simulink model "SF104A_MotCurrRegCfg"  (R2013b)
settings: Solver=FixedStepDiscrete  SolverMode=SingleTasking  StartTime=0.0  StopTime=1  FixedStep=0.002  RelTol=1e-3
values from neighbouring files (symbols this model uses):
  ARCHGLBPRM_2MILLISEC_SEC_F32 = DataDict.Constant    [SF104A_MotCurrRegCfg_DataDict.m]
  ARCHGLBPRM_2PI_ULS_F32 = DataDict.Constant    [SF104A_MotCurrRegCfg_DataDict.m]
  ARCHGLBPRM_HALFSQRT3_ULS_F32 = DataDict.Constant    [SF104A_MotCurrRegCfg_DataDict.m]
  MotCurrRegCfgCtrlrDynGainVehSpdCutOff = DataDict.Calibration    [SF104A_MotCurrRegCfg_DataDict.m]
  MotCurrRegCfgCurrLoopSecOrderTrfFctEna = DataDict.Calibration    [SF104A_MotCurrRegCfg_DataDict.m]
  MotCurrRegCfgIntglGainSampleTi = DataDict.Calibration    [SF104A_MotCurrRegCfg_DataDict.m]
  MotCurrRegCfgMotAgCompuDly = DataDict.Calibration    [SF104A_MotCurrRegCfg_DataDict.m]
  MotCurrRegCfgMotClsdLoopBwDaxY = DataDict.Calibration    [SF104A_MotCurrRegCfg_DataDict.m]
  MotCurrRegCfgMotClsdLoopBwQaxY = DataDict.Calibration    [SF104A_MotCurrRegCfg_DataDict.m]
  MotCurrRegCfgMotDampgRatDax = DataDict.Calibration    [SF104A_MotCurrRegCfg_DataDict.m]
  MotCurrRegCfgMotDampgRatQax = DataDict.Calibration    [SF104A_MotCurrRegCfg_DataDict.m]
  MotCurrRegCfgMotNatFrqDaxY = DataDict.Calibration    [SF104A_MotCurrRegCfg_DataDict.m]
  MotCurrRegCfgMotNatFrqQaxY = DataDict.Calibration    [SF104A_MotCurrRegCfg_DataDict.m]
  MotCurrRegCfgMotRVirtDax = DataDict.Calibration    [SF104A_MotCurrRegCfg_DataDict.m]
  MotCurrRegCfgMotRVirtQax = DataDict.Calibration    [SF104A_MotCurrRegCfg_DataDict.m]
  MOTDAMPGRATCON_ULS_F32 = DataDict.Constant    [SF104A_MotCurrRegCfg_DataDict.m]
  MotRefMdlFbCtrlDi = DataDict.ImprtdCal    [SF104A_MotCurrRegCfg_DataDict.m]
  POLETOPHA_ULS_F32 = DataDict.Constant    [SF104A_MotCurrRegCfg_DataDict.m]
  SysGlbPrmMotPoleCnt = DataDict.ImprtdCal    [SF104A_MotCurrRegCfg_DataDict.m]
  ZEROMOTCTRLGAIN_OHM_F32 = DataDict.Constant    [SF104A_MotCurrRegCfg_DataDict.m]
undefined symbols (not defined in the file or in its folder): MotCurrEolCalSt2
libraries: NxtrLim x11, FixdToFloat x4, LnrIntrpn x4, simulink x3, Fil x2, FloatToFixd x1
(part 1 of 3)
settings Model: Creator=qzwc4r  LastModifiedBy=RZ2YLP
settings SolverCC: AutoInsertRateTranBlk=on  InsertRTBMode=Always
settings DataIOCC: LimitDataPoints=off  SaveFormat=Structure  ReturnWorkspaceOutputs=on
settings OptimizationCC: BlockReduction=off  InlineParams=on  ZeroExternalMemoryAtStartup=off  ZeroInternalMemoryAtStartup=off  OptimizeModelRefInitCode=on  LifeSpan=1
settings DebuggingCC: SignalInfNanChecking=error  SignalRangeChecking=warning  UnderspecifiedInitializationDetection=Simplified  SolverPrmCheckMsg=error  InheritedTsInSrcMsg=error  DiscreteInheritContinuousMsg=error  SingleTaskRateTransMsg=error  TasksWithSamePriorityMsg=error  SigSpecEnsureSampleTimeMsg=error  CheckMatrixSingularityMsg=error  ParameterUnderflowMsg=error  ParameterPrecisionLossMsg=error  ParameterTunabilityLossMsg=error  FixptConstUnderflowMsg=warning  FixptConstOverflowMsg=warning  VectorMatrixConversionMsg=error  SignalLabelMismatchMsg=error  UnconnectedInputMsg=error  UnconnectedOutputMsg=error  UnconnectedLineMsg=error  SFcnCompatibilityMsg=error  UniqueDataStoreMsg=warning  BusObjectLabelMismatch=error  RootOutportRequireBusObject=error  AssertControl=DisableAll  ModelReferenceIOMsg=error  ModelReferenceVersionMismatchMessage=warning  ModelReferenceIOMismatchMessage=error  ModelReferenceCSMismatchMessage=warning  ModelReferenceDataLoggingMessage=error  StateNameClashWarn=warning  StrictBusMsg=ErrorOnBusTreatedAsVector  NonBusSignalsTreatedAsBus=error  SFUnexpectedBacktrackingDiag=error  SFInvalidInputDataAccessInChartInitDiag=error  SFNoUnconditionalDefaultTransitionDiag=error  SFTransitionOutsideNaturalParentDiag=error  SFUnconditionalTransitionShadowingDiag=error  SFUndirectedBroadcastEventsDiag=error
settings ModelReferenceCC: ModelReferenceNumInstancesAllowed=Single
settings RTWCC: SystemTargetFile=autosar.tlc  GenCodeOnly=on  TemplateMakefile=ert_default_tmf  Description=AUTOSAR  GenerateReport=on  ProcessScript=autosar_make_rtw_hook  LaunchReport=on
settings CodeAppCC: GenerateComments=off  IgnoreCustomStorageClasses=off  CustomSymbolStrType=$N$R$M  CustomSymbolStrBlkIO=$N$M  SimulinkBlockComments=off
settings STFCustomTargetCC: ParMdlRefBuildCompliant=on  CompOptLevelCompliant=on  IncludeMdlTerminateFcn=off  CombineOutputUpdateFcns=on  SuppressErrorStatus=on  ERTFirstTimeCompliant=on  ERTCustomFileBanners=on  SupportNonFinite=off  SupportComplex=off  SupportContinuousTime=off  SupportNonInlinedSFcns=off  MATLABClassNameForMDSCustomization=Simulink.SoftwareTarget.ERTCustomization  AutosarCompliant=on  GRTInterface=off  SystemTargetFile=autosar.tlc
settings ERTTargetCC: CodeReplacementLibrary=ANSI_C  ConcurrentExecutionCompliant=off  IncludeMdlTerminateFcn=off  SuppressErrorStatus=on  SupportNonFinite=off  SupportComplex=off  ModelStepFunctionPrototypeControlCompliant=off  CPPClassGenCompliant=off  AutosarCompliant=on  InlinedParameterPlacement=NonHierarchical  ERTCustomFileTemplate=example_file_process.tlc  EnableUserReplacementTypes=on

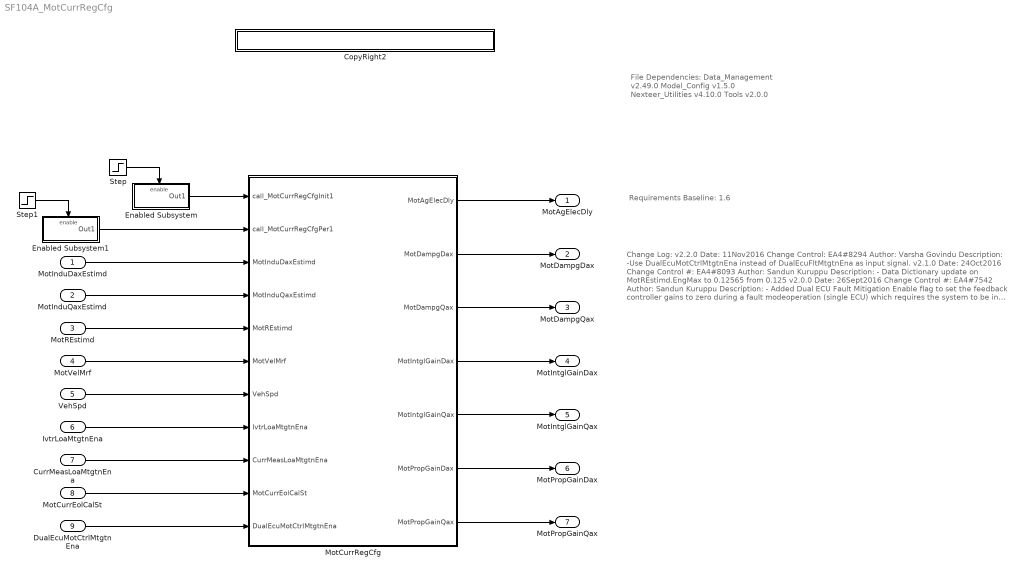
== system SF104A_MotCurrRegCfg ==
  note: File Dependencies:
      |
      | Data_Management v2.49.0
      | Model_Config v1.5.0
      | Nexteer_Utilities v4.10.0
      | Tools v2.0.0
  note: Requirements Baseline: 1.6
  note: Change Log:
      | v2.2.0
      | Date: 11Nov2016
      | Change Control: EA4#8294
      | Author: Varsha Govindu
      | Description:
      | -Use DualEcuMotCtrlMtgtnEna instead of DualEcuFltMtgtnEna as input signal.
      |
      | v2.1.0
      | Date: 24Oct2016
      | Change Control #: EA4#8093
      | Author: Sandun Kuruppu
      | Description:
      |  - Data Dictionary update on MotREstimd.EngMax to 0.12565 from 0.125
      |
      | v2.0.0
      | Date: 26Sept2016
      | Change Control #: EA4#7542
      | Author: Sandun Kuruppu
      | Description:
      | - Added Dual ECU Fault Mitigation Enable flag to set the feedback controller gains to
      | zero during a fault modeoperation (single ECU) which requires the system to be in feedforward
      | control mode
      |
      | v1.5.0
      | Date: 06Jun2016
      | Change Control #: EA4#6007
      | Author: Siva
      | Description:
      | - Updated the test tolerance value of 'MotIntglGainQax' and
      |    'MotIntglGainDax' from '1.49e-8' to '1.49e-7'.
      |
      |
      | v1.4.1
      | Date: 29April2016
      | Change Control #: EA4#5365
      | Author:  Siva
      | Description:
      | - HIghlighted only those blocks related to v1.4.0
      |
      |
      | v1.4.0
      | Date: 29April2016
      | Change Control #: EA4#5365
      | Author:  Siva
      | Description:
      | - Input signal name changed from 'MotCurrLoaMtgtnEna' to 'CurrMeasLoaMtgtnEna'.
      |
      |
      | v1.3.0
      | Date: 16November2015
      | Change Control #: EA4#2462
      | Author:  Fei Yuan
      | Description:
      | - Change MotCurrRegCfgMotClsdLoopBwDaxY.EngMax to 1000 and chagne
      |   MotCurrRegCfgMotNatFrqQaxY.EngMax to 500.
      | - Add dependencies "MotRefMdl","SysGlbPrm", "ArchGlbPrm".
      | - Correct the abbreviations which were not in the key word list,
      |   MotCurrRegCfgCurrLoopSecOrderTrfFctEna, MotCurrRegCfgIntglGainSampleTi
      |   and MotCurrRegCfgMotCtrlPrmSeInx.
      | - Add Header "ArchGlbPrm" and chagne Define to "Global" for the global constants
      |   ARCHGLBPRM_2MILLISEC_SEC_F32, ARCHGLBPRM_2PI_ULS_F32 and
      |   ARCHGLBPRM_HALFSQRT3_ULS_F32
      | - Add 2 constants POLETOPHA_ULS_F32 and MOTDAMPGRATCON_ULS_F32 to
      |   avoid "magic" numbers
      |
      | v1.2.0
      | Date: 17June2015
      | Change Control #:  EA4#772
      | DRW:  Kevin Derry
      | Description:
      | - IF logic simplified in Feedback_Control_Enabled.
      | - Redundant FixdToFloat blocks eliminated by moving after Merge blocks.
      | - Changed Max blocks to Width and Selector blocks in Feedback_Control_ Enabled.
      | - Added two more zero-outputs from Feedback_Control_Disabled block.
      | - Use_Lookup_Table now has just one FloatToFixd block placed before branching.
      |
      |
      | v1.1.0
      | Date 15June2015
      | Change Control #: EA4#772
      | DRW: K Derry
      | Description:
      | - Reduced number of decimal points used in EngMin and EngMax
      |   of MotCurrRegCfgIntgrlGainSampleTi calibration.
      | - Changed PortName of  MotCurrRegCfgMotClsdLoopBwDaxY
      |   from 'UNDEFINED' to its own name.
      | - Changed EngDT from u5p11 to float32 for MotCurrRegCfgMotDampgRatDax
      |   and MotCurrRegCfgMotDampgRatQax.
      | - In model, set MotVelMrfFild memory block's diagnsitcs to "None" to prevent
      |   runtime warnings.
      | - Renamed block from MotCurrRegCfgInit to MotCurrRegCfgInit1.
      |
      | v1.0.0
      | Date: 05June2015
      | Change Control #: EA4#291
      | DRW: P. Lefler
      | Description:
      | - Initial Release
  MotInduDaxEstimd : Inport  RequirementInfo={} %GIDa_f2a3713f_af81_4fac_b34d_14f3e5e1b0be
  MotInduQaxEstimd : Inport  RequirementInfo={} %GIDa_499434ce_4059_49ae_8df4_5a3d844745e5  Port=2
  MotREstimd : Inport  RequirementInfo={} %GIDa_613252af_40b2_4cf8_bf58_b3cc68c1c009  Port=3
  MotVelMrf : Inport  RequirementInfo={} %GIDa_322039a3_e6fe_42bc_aa12_8e24eb17e2f4  Port=4
  VehSpd : Inport  RequirementInfo={} %GIDa_fa3348f2_b626_4aad_a658_f6996eb2def3  Port=5
  IvtrLoaMtgtnEna : Inport  RequirementInfo={} %GIDa_2d274148_1bc4_42fc_ab0a_2f934c9b59fb  Port=6
  CurrMeasLoaMtgtnEna : Inport  RequirementInfo={} %GIDa_fed047b5_6986_4faf_9f83_25b4cca19370  Port=7
  MotCurrEolCalSt : Inport  RequirementInfo={} %GIDa_32d8f749_6a45_4e42_adc8_ac0d93f6ae86  Port=8
  DualEcuMotCtrlMtgtnEna : Inport  RequirementInfo={} %GIDa_c76bf203_6df8_416a_9b83_0ec7df30f445  Port=9
  CopyRight2 : Subsystem  Description=|  mask(Copyright Information){none=on}
      | Copyright info block.                                               
      |                                                                     
      | Place copyright information at the top of every subsystem in design.
      mask prompts: none "No parameters"
      mask help: Place copyright information at the top of every subsystem in design.
      mask Display:
      | NxtrConf = 'Nexteer Confidential';
      | 
      | sys = bdroot; %handle for the current model ("system")
      | first = get_param(sys,'Created');
      | if(isempty(first))
      |     first = datestr(now,'yyyy');
      | else
      |     first = first(end-3:end);  %year is last four digits
      | end
      | 
      | last = get_param(sys,'LastModifiedDate');
      | if isempty(last)
      |     last = datestr(now,'yyyy');
      | else
      |     last = last(end-3:end);
      | end
      | 
      | if strcmp(first,last)
      |     fprintf('%s -- Copyright %s Nexteer',NxtrConf,first)
      | else
      |     fprintf('%s -- %s%s- %s Nexteer',NxtrConf,char(169),first,last)
      | end
  Enabled Subsystem : Subsystem  RequirementInfo={} %GIDa_effa6e24_8ba6_4497_9db0_85737a800e07  TreatAsAtomicUnit=on
  Enabled Subsystem1 : Subsystem  RequirementInfo={} %GIDa_1bee6874_e426_4288_bd8a_5516be879145  TreatAsAtomicUnit=on
  MotCurrRegCfg : Subsystem  RequirementInfo={} %GIDa_30303013_0275_4f3e_a6a9_9715e2a59d99
      settings: AttributesFormatString=%<Tag>
  Step : Step  RequirementInfo={} %GIDa_f21df76b_ca1d_45ef_b333_d26310ef5ed0  Time=.00001  Before=1  After=0  SampleTime=0.002
  Step1 : Step  RequirementInfo={} %GIDa_c05f0e21_f7b5_43d6_b3e6_918200909a8d  Time=.00001  SampleTime=0.002
  MotAgElecDly : Outport  RequirementInfo={} %GIDa_0001b80f_658e_468d_9e3b_e8dd3d1e87d9
  MotDampgDax : Outport  RequirementInfo={} %GIDa_7ba8811f_575e_45a3_b9ab_c9a20ded865a  Port=2
  MotDampgQax : Outport  RequirementInfo={} %GIDa_21431bb9_1b91_45e4_9edb_ea1e11969312  Port=3
  MotIntglGainDax : Outport  RequirementInfo={} %GIDa_a0075132_5a25_47b2_a9d5_e71863c4bc1d  Port=4
  MotIntglGainQax : Outport  RequirementInfo={} %GIDa_3e60d556_d18f_463b_920f_433ffe998fc6  Port=5
  MotPropGainDax : Outport  RequirementInfo={} %GIDa_84dec573_fa64_4c43_87c4_5739341b195f  Port=6
  MotPropGainQax : Outport  RequirementInfo={} %GIDa_04cf0d55_14aa_4fa9_ad4e_46d8ac433649  Port=7
  wires:
  MotInduDaxEstimd/1 -> MotCurrRegCfg/3(MotInduDaxEstimd)
  MotInduQaxEstimd/1 -> MotCurrRegCfg/4(MotInduQaxEstimd)
  MotREstimd/1 -> MotCurrRegCfg/5(MotREstimd)
  MotVelMrf/1 -> MotCurrRegCfg/6(MotVelMrf)
  VehSpd/1 -> MotCurrRegCfg/7(VehSpd)
  IvtrLoaMtgtnEna/1 -> MotCurrRegCfg/8(IvtrLoaMtgtnEna)
  CurrMeasLoaMtgtnEna/1 -> MotCurrRegCfg/9(CurrMeasLoaMtgtnEna)
  MotCurrEolCalSt/1 -> MotCurrRegCfg/10(MotCurrEolCalSt)
  MotCurrRegCfg/1(MotAgElecDly) -> MotAgElecDly/1
  MotCurrRegCfg/2(MotDampgDax) -> MotDampgDax/1
  MotCurrRegCfg/3(MotDampgQax) -> MotDampgQax/1
  MotCurrRegCfg/4(MotIntglGainDax) -> MotIntglGainDax/1
  MotCurrRegCfg/5(MotIntglGainQax) -> MotIntglGainQax/1
  MotCurrRegCfg/6(MotPropGainDax) -> MotPropGainDax/1
  MotCurrRegCfg/7(MotPropGainQax) -> MotPropGainQax/1
  DualEcuMotCtrlMtgtnEna/1 -> MotCurrRegCfg/11(DualEcuMotCtrlMtgtnEna)
  Enabled Subsystem1/1(Out1) -> MotCurrRegCfg/2(call_MotCurrRegCfgPer1)
  Enabled Subsystem/1(Out1) -> MotCurrRegCfg/1(call_MotCurrRegCfgInit1)
  Step/1 -> Enabled Subsystem/Enable
  Step1/1 -> Enabled Subsystem1/Enable

== system SF104A_MotCurrRegCfg/CopyRight2 ==

== system SF104A_MotCurrRegCfg/Enabled Subsystem ==
  Enable : EnablePort
  Function-Call Generator : simulink/Ports & Subsystems/Function-Call Generator  sample_time=.002  numberOfIterations=1
  Out1 : Outport
  wires:
  Function-Call Generator/1 -> Out1/1

== system SF104A_MotCurrRegCfg/Enabled Subsystem1 ==
  Enable : EnablePort
  Function-Call Generator : simulink/Ports & Subsystems/Function-Call Generator  sample_time=.002  numberOfIterations=1
  Out1 : Outport
  wires:
  Function-Call Generator/1 -> Out1/1

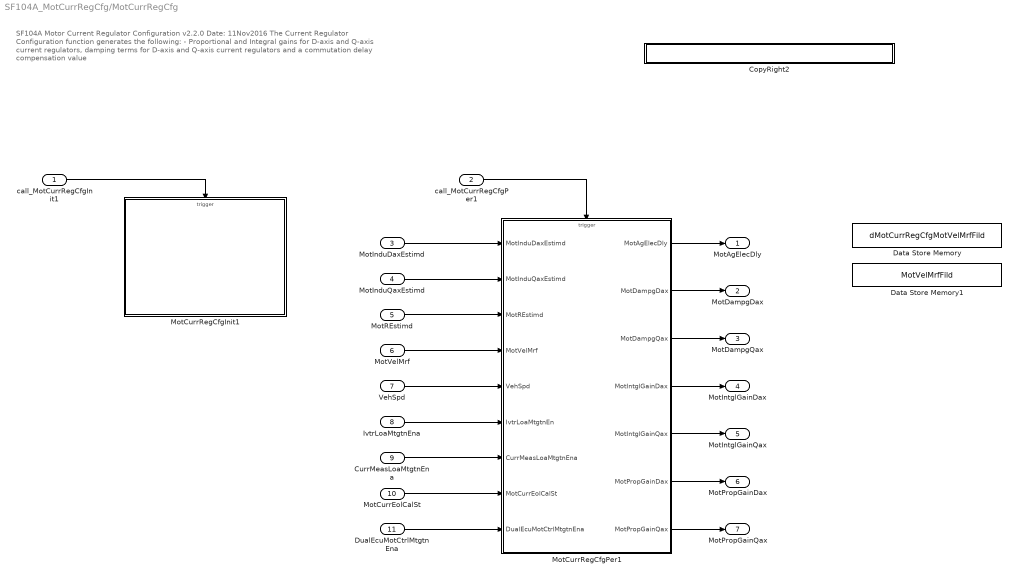
== system SF104A_MotCurrRegCfg/MotCurrRegCfg ==
  note: SF104A  Motor Current Regulator Configuration
      | v2.2.0
      | Date: 11Nov2016
      |
      | The Current Regulator Configuration function generates the following:
      |    - Proportional and Integral gains for D-axis and Q-axis current regulators,
      |     damping terms for D-axis and Q-axis current regulators and a commutation delay compensation value
  call_MotCurrRegCfgInit1 : Inport  RequirementInfo={} %GIDa_89b8ee72_a07a_46f4_939f_d05bf9b2c2f6
  call_MotCurrRegCfgPer1 : Inport  Port=2
  MotInduDaxEstimd : Inport  RequirementInfo="{'linktype_rmi_doors' '0000bb43 (/E-STEER Core/SubSystem Specifications/Application Functions/SF99/SF104A Current Regulator Configuration)' '#SF104A_46' 'true' 'REQ:  SF104A_46' '' } %GIDa_8d89b146_391a_4304_b17d_54d974ce8e05"  Port=3
  MotInduQaxEstimd : Inport  RequirementInfo="{'linktype_rmi_doors' '0000bb43 (/E-STEER Core/SubSystem Specifications/Application Functions/SF99/SF104A Current Regulator Configuration)' '#SF104A_47' 'true' 'REQ:  SF104A_47' '' } %GIDa_5a2f0e84_abeb_44bc_a9c7_1a1aa0b41f91"  Port=4
  MotREstimd : Inport  RequirementInfo="{'linktype_rmi_doors' '0000bb43 (/E-STEER Core/SubSystem Specifications/Application Functions/SF99/SF104A Current Regulator Configuration)' '#SF104A_45' 'true' 'REQ:  SF104A_45' '' } %GIDa_eb069174_7e58_4262_92bf_396541a51772"  Port=5
  MotVelMrf : Inport  RequirementInfo="{'linktype_rmi_doors' '0000bb43 (/E-STEER Core/SubSystem Specifications/Application Functions/SF99/SF104A Current Regulator Configuration)' '#SF104A_27' 'true' 'REQ:  SF104A_27' '' } %GIDa_4f9a3fc7_c710_4be4_b23d_f1cddddea8a3"  Port=6
  VehSpd : Inport  RequirementInfo="{'linktype_rmi_doors' '0000bb43 (/E-STEER Core/SubSystem Specifications/Application Functions/SF99/SF104A Current Regulator Configuration)' '#SF104A_43' 'true' 'REQ:  SF104A_43' '' } %GIDa_0630ae4e_95ba_462c_9688_e21f36c9e958"  Port=7
  IvtrLoaMtgtnEna : Inport  RequirementInfo="{'linktype_rmi_doors' '0000bb43 (/E-STEER Core/SubSystem Specifications/Application Functions/SF99/SF104A Current Regulator Configuration)' '#SF104A_120' 'true' 'REQ:  SF104A_120' '' } %GIDa_f0741086_1bc8_4a8f_8784_a68ec8bc7278"  Port=8
  CurrMeasLoaMtgtnEna : Inport  RequirementInfo="{'linktype_rmi_doors' '0000bb43 (/E-STEER Core/SubSystem Specifications/Application Functions/SF99/SF104A Current Regulator Configuration)' '#SF104A_119' 'true' 'REQ:  SF104A_119' '' } %GIDa_4c4ca071_2cf4_4bb5_8575_605f49228235"  Port=9
  MotCurrEolCalSt : Inport  RequirementInfo="{'linktype_rmi_doors' '0000bb43 (/E-STEER Core/SubSystem Specifications/Application Functions/SF99/SF104A Current Regulator Configuration)' '#SF104A_44' 'true' 'REQ:  SF104A_44' '' } %GIDa_92e78dc8_c2f9_49ab_a345_7a0326158378"  Port=10
  DualEcuMotCtrlMtgtnEna : Inport  RequirementInfo="{'linktype_rmi_doors' '0000bb43 (/E-STEER Core/SubSystem Specifications/Application Functions/SF99/SF104A Current Regulator Configuration)' '#SF104A_126' 'true' 'REQ:  SF104A_126' '' } %GIDa_47c60167_79be_4b75_9326_1776d0cf72bf"  Port=11
  CopyRight2 : Subsystem  Description=|  mask(Copyright Information){none=on}
      | Copyright info block.                                               
      |                                                                     
      | Place copyright information at the top of every subsystem in design.
      mask prompts: none "No parameters"
      mask help: Place copyright information at the top of every subsystem in design.
      mask Display:
      | NxtrConf = 'Nexteer Confidential';
      | 
      | sys = bdroot; %handle for the current model ("system")
      | first = get_param(sys,'Created');
      | if(isempty(first))
      |     first = datestr(now,'yyyy');
      | else
      |     first = first(end-3:end);  %year is last four digits
      | end
      | 
      | last = get_param(sys,'LastModifiedDate');
      | if isempty(last)
      |     last = datestr(now,'yyyy');
      | else
      |     last = last(end-3:end);
      | end
      | 
      | if strcmp(first,last)
      |     fprintf('%s -- Copyright %s Nexteer',NxtrConf,first)
      | else
      |     fprintf('%s -- %s%s- %s Nexteer',NxtrConf,char(169),first,last)
      | end
  Data Store Memory : DataStoreMemory  DataStoreName=dMotCurrRegCfgMotVelMrfFild  ReadBeforeWriteMsg=warning  WriteAfterWriteMsg=warning  WriteAfterReadMsg=warning  StateMustResolveToSignalObject=on
  Data Store Memory1 : DataStoreMemory  RequirementInfo="{'linktype_rmi_doors' '0000bb43 (/E-STEER Core/SubSystem Specifications/Application Functions/SF99/SF104A Current Regulator Configuration)' '#SF104A_57' 'true' 'REQ:  SF104A_57' '' } %GIDa_2816ad37_1dd8_467d_a813_ae50490bafd5"  DataStoreName=MotVelMrfFild  InitialValue=[]  StateMustResolveToSignalObject=on
  MotCurrRegCfgInit1 : Subsystem  TreatAsAtomicUnit=on
  MotCurrRegCfgPer1 : Subsystem  TreatAsAtomicUnit=on
  MotAgElecDly : Outport  RequirementInfo="{'linktype_rmi_doors' '0000bb43 (/E-STEER Core/SubSystem Specifications/Application Functions/SF99/SF104A Current Regulator Configuration)' '#SF104A_55' 'true' 'REQ:  SF104A_55' '' } %GIDa_43076b25_8e32_4349_8562_0121bc0cf86e"
  MotDampgDax : Outport  RequirementInfo="{'linktype_rmi_doors' '0000bb43 (/E-STEER Core/SubSystem Specifications/Application Functions/SF99/SF104A Current Regulator Configuration)' '#SF104A_53' 'true' 'REQ:  SF104A_53' '' } %GIDa_7a762bc6_7e48_4bbf_bf24_9dc61dc71eb7"  Port=2
  MotDampgQax : Outport  RequirementInfo="{'linktype_rmi_doors' '0000bb43 (/E-STEER Core/SubSystem Specifications/Application Functions/SF99/SF104A Current Regulator Configuration)' '#SF104A_54' 'true' 'REQ:  SF104A_54' '' } %GIDa_4e4775a3_f5ea_4c13_8c68_5d0d7d55ff2d"  Port=3
  MotIntglGainDax : Outport  RequirementInfo="{'linktype_rmi_doors' '0000bb43 (/E-STEER Core/SubSystem Specifications/Application Functions/SF99/SF104A Current Regulator Configuration)' '#SF104A_51' 'true' 'REQ:  SF104A_51' '' } %GIDa_ad559d2d_2f69_47f7_97da_9be948795139"  Port=4
  MotIntglGainQax : Outport  RequirementInfo="{'linktype_rmi_doors' '0000bb43 (/E-STEER Core/SubSystem Specifications/Application Functions/SF99/SF104A Current Regulator Configuration)' '#SF104A_52' 'true' 'REQ:  SF104A_52' '' } %GIDa_7257c583_4b43_4ee6_acf5_24f02908af3f"  Port=5
  MotPropGainDax : Outport  RequirementInfo="{'linktype_rmi_doors' '0000bb43 (/E-STEER Core/SubSystem Specifications/Application Functions/SF99/SF104A Current Regulator Configuration)' '#SF104A_28' 'true' 'REQ:  SF104A_28' '' } %GIDa_504772d2_d87c_467b_98a8_df8457c8e1c6"  Port=6
  MotPropGainQax : Outport  RequirementInfo="{'linktype_rmi_doors' '0000bb43 (/E-STEER Core/SubSystem Specifications/Application Functions/SF99/SF104A Current Regulator Configuration)' '#SF104A_49' 'true' 'REQ:  SF104A_49' '' } %GIDa_bc54d691_d90c_4464_a2e3_c53440246af7"  Port=7
  wires:
  call_MotCurrRegCfgInit1/1 -> MotCurrRegCfgInit1/Trigger
  call_MotCurrRegCfgPer1/1 -> MotCurrRegCfgPer1/Trigger
  MotInduDaxEstimd/1 -> MotCurrRegCfgPer1/1(MotInduDaxEstimd)
  MotInduQaxEstimd/1 -> MotCurrRegCfgPer1/2(MotInduQaxEstimd)
  MotREstimd/1 -> MotCurrRegCfgPer1/3(MotREstimd)
  MotVelMrf/1 -> MotCurrRegCfgPer1/4(MotVelMrf)
  VehSpd/1 -> MotCurrRegCfgPer1/5(VehSpd)
  MotCurrRegCfgPer1/1(MotAgElecDly) -> MotAgElecDly/1
  MotCurrRegCfgPer1/2(MotDampgDax) -> MotDampgDax/1
  MotCurrRegCfgPer1/3(MotDampgQax) -> MotDampgQax/1
  MotCurrRegCfgPer1/4(MotIntglGainDax) -> MotIntglGainDax/1
  MotCurrRegCfgPer1/5(MotIntglGainQax) -> MotIntglGainQax/1
  MotCurrRegCfgPer1/6(MotPropGainDax) -> MotPropGainDax/1
  MotCurrRegCfgPer1/7(MotPropGainQax) -> MotPropGainQax/1
  IvtrLoaMtgtnEna/1 -> MotCurrRegCfgPer1/6(IvtrLoaMtgtnEn)
  CurrMeasLoaMtgtnEna/1 -> MotCurrRegCfgPer1/7(CurrMeasLoaMtgtnEna)
  MotCurrEolCalSt/1 -> MotCurrRegCfgPer1/8(MotCurrEolCalSt)
  DualEcuMotCtrlMtgtnEna/1 -> MotCurrRegCfgPer1/9(DualEcuMotCtrlMtgtnEna)

== system SF104A_MotCurrRegCfg/MotCurrRegCfg/CopyRight2 ==

== system SF104A_MotCurrRegCfg/MotCurrRegCfg/MotCurrRegCfgInit1 ==
  function : TriggerPort  TriggerType=function-call
  CopyRight2 : Subsystem  Description=|  mask(Copyright Information){none=on}
      | Copyright info block.                                               
      |                                                                     
      | Place copyright information at the top of every subsystem in design.
      mask prompts: none "No parameters"
      mask help: Place copyright information at the top of every subsystem in design.
      mask Display:
      | NxtrConf = 'Nexteer Confidential';
      | 
      | sys = bdroot; %handle for the current model ("system")
      | first = get_param(sys,'Created');
      | if(isempty(first))
      |     first = datestr(now,'yyyy');
      | else
      |     first = first(end-3:end);  %year is last four digits
      | end
      | 
      | last = get_param(sys,'LastModifiedDate');
      | if isempty(last)
      |     last = datestr(now,'yyyy');
      | else
      |     last = last(end-3:end);
      | end
      | 
      | if strcmp(first,last)
      |     fprintf('%s -- Copyright %s Nexteer',NxtrConf,first)
      | else
      |     fprintf('%s -- %s%s- %s Nexteer',NxtrConf,char(169),first,last)
      | end
  FilLpInit : Fil/FilLpInit  RequirementInfo="{'linktype_rmi_doors' '0000bb43 (/E-STEER Core/SubSystem Specifications/Application Functions/SF99/SF104A Current Regulator Configuration)' '#SF104A_62' 'true' 'REQ:  SF104A_62' '' } %GIDa_c6961b9d_0154_4477_9ad8_9e34eb942fcb"  Ic=0  Ts=ARCHGLBPRM_2MILLISEC_SEC_F32  Freq=MotCurrRegCfgMotVelFilFrq  StVar=MotVelMrfFild

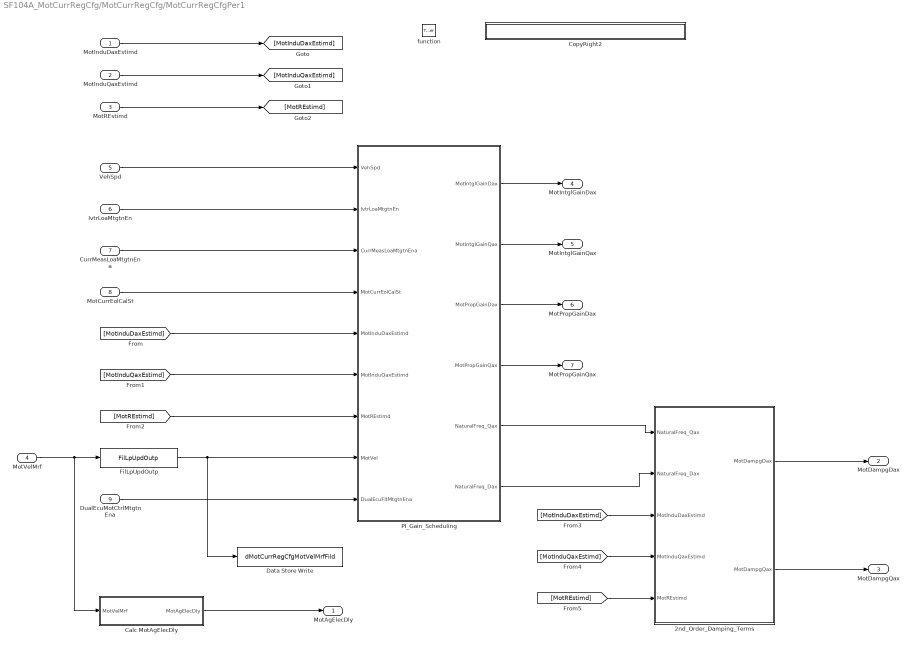
== system SF104A_MotCurrRegCfg/MotCurrRegCfg/MotCurrRegCfgPer1 ==
  MotInduDaxEstimd : Inport
  MotInduQaxEstimd : Inport  Port=2
  MotREstimd : Inport  Port=3
  MotVelMrf : Inport  Port=4
  VehSpd : Inport  Port=5
  IvtrLoaMtgtnEn : Inport  Port=6
  CurrMeasLoaMtgtnEna : Inport  Port=7
  MotCurrEolCalSt : Inport  Port=8
  DualEcuMotCtrlMtgtnEna : Inport  RequirementInfo="{'linktype_rmi_doors' '0000bb43 (/E-STEER Core/SubSystem Specifications/Application Functions/SF99/SF104A Current Regulator Configuration)' '#SF104A_44' 'true' 'REQ:  SF104A_44' '' } %GIDa_70157092_0448_4861_8c8d_842236aa4472"  Port=9
  function : TriggerPort  TriggerType=function-call
  2nd_Order_Damping_Terms : Subsystem  RequirementInfo="{'linktype_rmi_doors' '0000bb43 (/E-STEER Core/SubSystem Specifications/Application Functions/SF99/SF104A Current Regulator Configuration)' '#SF104A_74' 'true' 'REQ:  SF104A_74' '' } %GIDa_01b95588_6e5d_40a2_96e3_adc39de608fb"
  Calc MotAgElecDly : Subsystem  RequirementInfo="{'linktype_rmi_doors' '0000bb43 (/E-STEER Core/SubSystem Specifications/Application Functions/SF99/SF104A Current Regulator Configuration)' '#SF104A_94' 'true' 'REQ:  SF104A_94' '' } %GIDa_218ec898_1c8d_4425_b465_860fe3b3e0cb"
  CopyRight2 : Subsystem  Description=|  mask(Copyright Information){none=on}
      | Copyright info block.                                               
      |                                                                     
      | Place copyright information at the top of every subsystem in design.
      mask prompts: none "No parameters"
      mask help: Place copyright information at the top of every subsystem in design.
      mask Display:
      | NxtrConf = 'Nexteer Confidential';
      | 
      | sys = bdroot; %handle for the current model ("system")
      | first = get_param(sys,'Created');
      | if(isempty(first))
      |     first = datestr(now,'yyyy');
      | else
      |     first = first(end-3:end);  %year is last four digits
      | end
      | 
      | last = get_param(sys,'LastModifiedDate');
      | if isempty(last)
      |     last = datestr(now,'yyyy');
      | else
      |     last = last(end-3:end);
      | end
      | 
      | if strcmp(first,last)
      |     fprintf('%s -- Copyright %s Nexteer',NxtrConf,first)
      | else
      |     fprintf('%s -- %s%s- %s Nexteer',NxtrConf,char(169),first,last)
      | end
  Data Store Write : DataStoreWrite  DataStoreName=dMotCurrRegCfgMotVelMrfFild
  FilLpUpdOutp : Fil/FilLpUpdOutp  RequirementInfo="{'linktype_rmi_doors' '0000bb43 (/E-STEER Core/SubSystem Specifications/Application Functions/SF99/SF104A Current Regulator Configuration)' '#SF104A_57' 'true' 'REQ:  SF104A_57' '' } %GIDa_2429cc50_66f7_4688_89ce_0e31c2a15e8f"  StVar=MotVelMrfFild
      settings: AttributesFormatString=StVar: %<StVar>
  PI_Gain_Scheduling : Subsystem
  MotAgElecDly : Outport
  MotDampgDax : Outport  Port=2
  MotDampgQax : Outport  Port=3
  MotIntglGainDax : Outport  Port=4
  MotIntglGainQax : Outport  Port=5
  MotPropGainDax : Outport  Port=6
  MotPropGainQax : Outport  Port=7
  wires:
  MotVelMrf/1 -> Calc MotAgElecDly/1(MotVelMrf), FilLpUpdOutp/1
  Calc MotAgElecDly/1(MotAgElecDly) -> MotAgElecDly/1
  FilLpUpdOutp/1 -> Data Store Write/1, PI_Gain_Scheduling/8(MotVel)
  MotCurrEolCalSt/1 -> PI_Gain_Scheduling/4(MotCurrEolCalSt)
  CurrMeasLoaMtgtnEna/1 -> PI_Gain_Scheduling/3(CurrMeasLoaMtgtnEna)
  IvtrLoaMtgtnEn/1 -> PI_Gain_Scheduling/2(IvtrLoaMtgtnEn)
  VehSpd/1 -> PI_Gain_Scheduling/1(VehSpd)
  PI_Gain_Scheduling/1(MotIntglGainDax) -> MotIntglGainDax/1
  PI_Gain_Scheduling/2(MotIntglGainQax) -> MotIntglGainQax/1
  PI_Gain_Scheduling/3(MotPropGainDax) -> MotPropGainDax/1
  PI_Gain_Scheduling/4(MotPropGainQax) -> MotPropGainQax/1
  PI_Gain_Scheduling/5(NaturalFreq_Qax) -> 2nd_Order_Damping_Terms/1(NaturalFreq_Qax)
  PI_Gain_Scheduling/6(NaturalFreq_Dax) -> 2nd_Order_Damping_Terms/2(NaturalFreq_Dax)
  2nd_Order_Damping_Terms/1(MotDampgDax) -> MotDampgDax/1
  2nd_Order_Damping_Terms/2(MotDampgQax) -> MotDampgQax/1
  MotInduDaxEstimd/1 -> [MotInduDaxEstimd]
  MotInduQaxEstimd/1 -> [MotInduQaxEstimd]
  MotREstimd/1 -> [MotREstimd]
  [MotInduDaxEstimd] -> PI_Gain_Scheduling/5(MotInduDaxEstimd)
  [MotInduQaxEstimd] -> PI_Gain_Scheduling/6(MotInduQaxEstimd)
  [MotREstimd] -> PI_Gain_Scheduling/7(MotREstimd)
  [MotInduDaxEstimd] -> 2nd_Order_Damping_Terms/3(MotInduDaxEstimd)
  [MotInduQaxEstimd] -> 2nd_Order_Damping_Terms/4(MotInduQaxEstimd)
  [MotREstimd] -> 2nd_Order_Damping_Terms/5(MotREstimd)
  DualEcuMotCtrlMtgtnEna/1 -> PI_Gain_Scheduling/9(DualEcuFltMtgtnEna)

== system SF104A_MotCurrRegCfg/MotCurrRegCfg/MotCurrRegCfgInit1/CopyRight2 ==

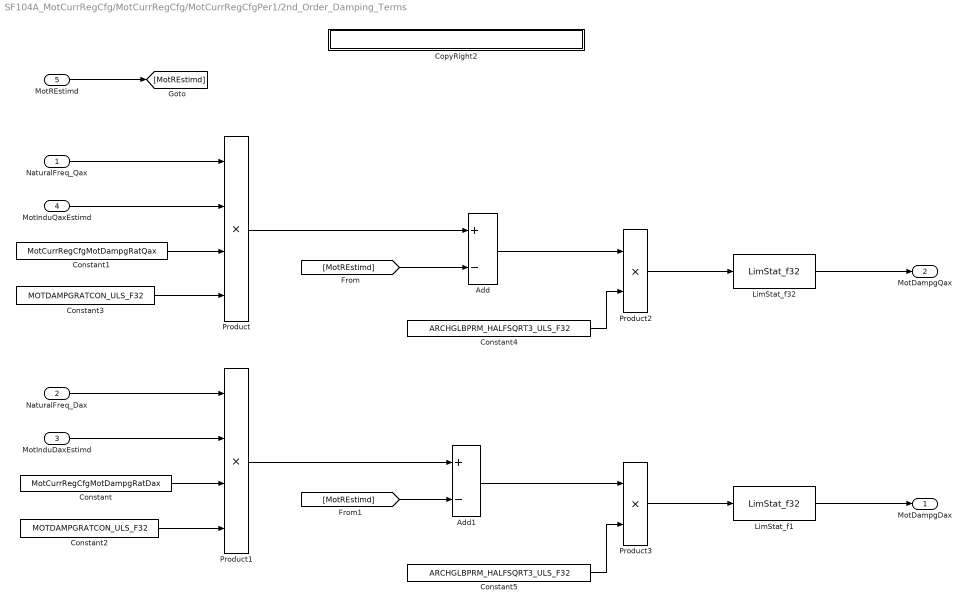
== system SF104A_MotCurrRegCfg/MotCurrRegCfg/MotCurrRegCfgPer1/2nd_Order_Damping_Terms ==
  NaturalFreq_Qax : Inport  RequirementInfo="{'linktype_rmi_doors' '0000bb43 (/E-STEER Core/SubSystem Specifications/Application Functions/SF99/SF104A Current Regulator Configuration)' '#SF104A_74' 'true' 'REQ:  SF104A_74' '' } %GIDa_d9e0da8f_3415_4633_aef8_b17d563eb7ee"
  NaturalFreq_Dax : Inport  RequirementInfo="{'linktype_rmi_doors' '0000bb43 (/E-STEER Core/SubSystem Specifications/Application Functions/SF99/SF104A Current Regulator Configuration)' '#SF104A_74' 'true' 'REQ:  SF104A_74' '' } %GIDa_233bb321_88e6_4330_a5fd_6f494bbd5c67"  Port=2
  MotInduDaxEstimd : Inport  RequirementInfo="{'linktype_rmi_doors' '0000bb43 (/E-STEER Core/SubSystem Specifications/Application Functions/SF99/SF104A Current Regulator Configuration)' '#SF104A_74' 'true' 'REQ:  SF104A_74' '' } %GIDa_459736c0_a51f_400e_bf95_5c4fc45ddc03"  Port=3
  MotInduQaxEstimd : Inport  RequirementInfo="{'linktype_rmi_doors' '0000bb43 (/E-STEER Core/SubSystem Specifications/Application Functions/SF99/SF104A Current Regulator Configuration)' '#SF104A_74' 'true' 'REQ:  SF104A_74' '' } %GIDa_b7ed7083_785a_4973_8a9e_384fb0c227a4"  Port=4
  MotREstimd : Inport  RequirementInfo="{'linktype_rmi_doors' '0000bb43 (/E-STEER Core/SubSystem Specifications/Application Functions/SF99/SF104A Current Regulator Configuration)' '#SF104A_74' 'true' 'REQ:  SF104A_74' '' } %GIDa_51d26aad_38c3_4145_b3b3_6d9618664903"  Port=5
  Add : Sum  RequirementInfo="{'linktype_rmi_doors' '0000bb43 (/E-STEER Core/SubSystem Specifications/Application Functions/SF99/SF104A Current Regulator Configuration)' '#SF104A_74' 'true' 'REQ:  SF104A_74' '' } %GIDa_d74664d5_cdfa_49db_b66d_915b8be5e5fa"  Inputs=+-
  Add1 : Sum  RequirementInfo="{'linktype_rmi_doors' '0000bb43 (/E-STEER Core/SubSystem Specifications/Application Functions/SF99/SF104A Current Regulator Configuration)' '#SF104A_74' 'true' 'REQ:  SF104A_74' '' } %GIDa_28004ede_8d47_4a3a_b118_c9381241ff52"  Inputs=+-
  Constant : Constant  RequirementInfo="{'linktype_rmi_doors' '0000bb43 (/E-STEER Core/SubSystem Specifications/Application Functions/SF99/SF104A Current Regulator Configuration)' '#SF104A_74' 'true' 'REQ:  SF104A_74' '' ; 'linktype_rmi_doors' '0000bb43 (/E-STEER Core/SubSystem Specifications/Application Functions/SF99/SF104A Current Regulator Configuration)' '#SF104A_71' 'true' 'REQ:  SF104A_71' '' } %GIDa_0c5c0ea0_b20b_4c5c_8d89_b9eeb7a26ae5"  Value=MotCurrRegCfgMotDampgRatDax
  Constant1 : Constant  RequirementInfo="{'linktype_rmi_doors' '0000bb43 (/E-STEER Core/SubSystem Specifications/Application Functions/SF99/SF104A Current Regulator Configuration)' '#SF104A_74' 'true' 'REQ:  SF104A_74' '' ; 'linktype_rmi_doors' '0000bb43 (/E-STEER Core/SubSystem Specifications/Application Functions/SF99/SF104A Current Regulator Configuration)' '#SF104A_71' 'true' 'REQ:  SF104A_71' '' } %GIDa_00bc6a83_c14c_48d2_a023_f3713efe60a2"  Value=MotCurrRegCfgMotDampgRatQax
  Constant2 : Constant  RequirementInfo="{'linktype_rmi_doors' '0000bb43 (/E-STEER Core/SubSystem Specifications/Application Functions/SF99/SF104A Current Regulator Configuration)' '#SF104A_74' 'true' 'REQ:  SF104A_74' '' } %GIDa_e1478153_67ed_436e_a516_cf58708f27be"  Value=MOTDAMPGRATCON_ULS_F32  OutDataTypeStr=single
  Constant3 : Constant  RequirementInfo="{'linktype_rmi_doors' '0000bb43 (/E-STEER Core/SubSystem Specifications/Application Functions/SF99/SF104A Current Regulator Configuration)' '#SF104A_74' 'true' 'REQ:  SF104A_74' '' } %GIDa_f365d753_2ce1_47bb_a3c8_b68433a7b8db"  Value=MOTDAMPGRATCON_ULS_F32  OutDataTypeStr=single
  Constant4 : Constant  RequirementInfo="{'linktype_rmi_doors' '0000bb43 (/E-STEER Core/SubSystem Specifications/Application Functions/SF99/SF104A Current Regulator Configuration)' '#SF104A_74' 'true' 'REQ:  SF104A_74' '' } %GIDa_f51c90c6_ebaf_425d_a03a_5a828cb16cf7"  Value=ARCHGLBPRM_HALFSQRT3_ULS_F32
  Constant5 : Constant  RequirementInfo="{'linktype_rmi_doors' '0000bb43 (/E-STEER Core/SubSystem Specifications/Application Functions/SF99/SF104A Current Regulator Configuration)' '#SF104A_74' 'true' 'REQ:  SF104A_74' '' } %GIDa_076d4432_d1d5_4b5c_a458_474be8e4d72b"  Value=ARCHGLBPRM_HALFSQRT3_ULS_F32
  CopyRight2 : Subsystem  Description=|  mask(Copyright Information){none=on}
      | Copyright info block.                                               
      |                                                                     
      | Place copyright information at the top of every subsystem in design.
      mask prompts: none "No parameters"
      mask help: Place copyright information at the top of every subsystem in design.
      mask Display:
      | NxtrConf = 'Nexteer Confidential';
      | 
      | sys = bdroot; %handle for the current model ("system")
      | first = get_param(sys,'Created');
      | if(isempty(first))
      |     first = datestr(now,'yyyy');
      | else
      |     first = first(end-3:end);  %year is last four digits
      | end
      | 
      | last = get_param(sys,'LastModifiedDate');
      | if isempty(last)
      |     last = datestr(now,'yyyy');
      | else
      |     last = last(end-3:end);
      | end
      | 
      | if strcmp(first,last)
      |     fprintf('%s -- Copyright %s Nexteer',NxtrConf,first)
      | else
      |     fprintf('%s -- %s%s- %s Nexteer',NxtrConf,char(169),first,last)
      | end
  LimStat_f1 : NxtrLim/LimStat_f32  RequirementInfo="{'linktype_rmi_doors' '0000bb43 (/E-STEER Core/SubSystem Specifications/Application Functions/SF99/SF104A Current Regulator Configuration)' '#SF104A_96' 'true' 'REQ:  SF104A_96' '' } %GIDa_b1b28976_b68b_4689_b326_bfd5a316d3fb"  LoLim=MOTDAMPGLOLIM_OHM_F32  HiLim=MOTDAMPGHILIM_OHM_F32
      settings: AttributesFormatString=|
      | Low Limit: %<LoLim>
      | High Limit:%<HiLim>
  LimStat_f32 : NxtrLim/LimStat_f32  RequirementInfo="{'linktype_rmi_doors' '0000bb43 (/E-STEER Core/SubSystem Specifications/Application Functions/SF99/SF104A Current Regulator Configuration)' '#SF104A_96' 'true' 'REQ:  SF104A_96' '' } %GIDa_efc703cd_7e72_41a4_90e4_b369c76bda41"  LoLim=MOTDAMPGLOLIM_OHM_F32  HiLim=MOTDAMPGHILIM_OHM_F32
      settings: AttributesFormatString=|
      | Low Limit: %<LoLim>
      | High Limit:%<HiLim>
  Product : Product  RequirementInfo="{'linktype_rmi_doors' '0000bb43 (/E-STEER Core/SubSystem Specifications/Application Functions/SF99/SF104A Current Regulator Configuration)' '#SF104A_74' 'true' 'REQ:  SF104A_74' '' } %GIDa_e2a14d79_7e1e_42b1_8049_3772d39898fd"  Inputs=4
  Product1 : Product  RequirementInfo="{'linktype_rmi_doors' '0000bb43 (/E-STEER Core/SubSystem Specifications/Application Functions/SF99/SF104A Current Regulator Configuration)' '#SF104A_74' 'true' 'REQ:  SF104A_74' '' } %GIDa_c6b31c08_c75a_4a9a_bbfe_d54350e8ca09"  Inputs=4
  Product2 : Product  RequirementInfo="{'linktype_rmi_doors' '0000bb43 (/E-STEER Core/SubSystem Specifications/Application Functions/SF99/SF104A Current Regulator Configuration)' '#SF104A_74' 'true' 'REQ:  SF104A_74' '' } %GIDa_aab3def3_47ac_48ad_8a7b_b9eec839bc42"
  Product3 : Product  RequirementInfo="{'linktype_rmi_doors' '0000bb43 (/E-STEER Core/SubSystem Specifications/Application Functions/SF99/SF104A Current Regulator Configuration)' '#SF104A_74' 'true' 'REQ:  SF104A_74' '' } %GIDa_b81216e2_90df_49c8_9deb_c92ea7700b3b"
  MotDampgDax : Outport  RequirementInfo="{'linktype_rmi_doors' '0000bb43 (/E-STEER Core/SubSystem Specifications/Application Functions/SF99/SF104A Current Regulator Configuration)' '#SF104A_74' 'true' 'REQ:  SF104A_74' '' } %GIDa_cc793281_3ab4_4039_942a_58c18ea1a110"
  MotDampgQax : Outport  RequirementInfo="{'linktype_rmi_doors' '0000bb43 (/E-STEER Core/SubSystem Specifications/Application Functions/SF99/SF104A Current Regulator Configuration)' '#SF104A_74' 'true' 'REQ:  SF104A_74' '' } %GIDa_c0917687_86db_4bcf_9d6b_15bce05bb6a2"  Port=2
  wires:
  NaturalFreq_Qax/1 -> Product/1
  MotInduQaxEstimd/1 -> Product/2
  Constant1/1 -> Product/3
  Constant3/1 -> Product/4
  NaturalFreq_Dax/1 -> Product1/1
  MotInduDaxEstimd/1 -> Product1/2
  Constant/1 -> Product1/3
  Constant2/1 -> Product1/4
  Product/1 -> Add/1
  MotREstimd/1 -> [MotREstimd]
  [MotREstimd] -> Add/2
  Product1/1 -> Add1/1
  [MotREstimd] -> Add1/2
  Add/1 -> Product2/1
  Add1/1 -> Product3/1
  Constant5/1 -> Product3/2
  Constant4/1 -> Product2/2
  Product3/1 -> LimStat_f1/1
  Product2/1 -> LimStat_f32/1
  LimStat_f32/1 -> MotDampgQax/1
  LimStat_f1/1 -> MotDampgDax/1

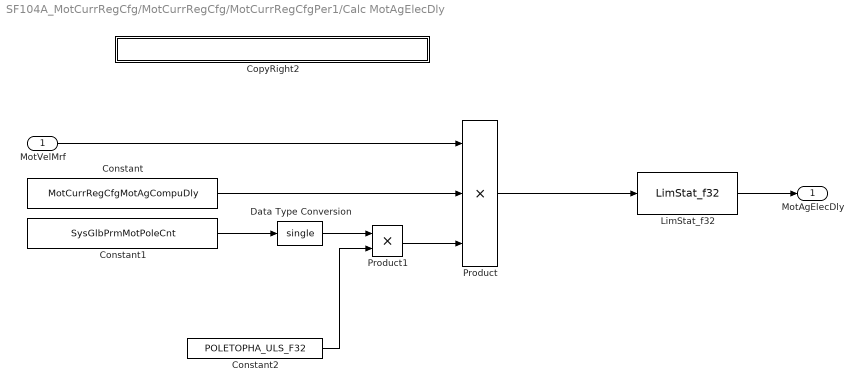
== system SF104A_MotCurrRegCfg/MotCurrRegCfg/MotCurrRegCfgPer1/Calc MotAgElecDly ==
  MotVelMrf : Inport  RequirementInfo="{'linktype_rmi_doors' '0000bb43 (/E-STEER Core/SubSystem Specifications/Application Functions/SF99/SF104A Current Regulator Configuration)' '#SF104A_95' 'true' 'REQ:  SF104A_95' '' } %GIDa_0629ad48_5a60_4f01_882f_abb1279b5eff"
  Constant : Constant  RequirementInfo="{'linktype_rmi_doors' '0000bb43 (/E-STEER Core/SubSystem Specifications/Application Functions/SF99/SF104A Current Regulator Configuration)' '#SF104A_95' 'true' 'REQ:  SF104A_95' '' } %GIDa_f598f786_29a4_4e6e_a848_03d8c2d6da6e"  Value=MotCurrRegCfgMotAgCompuDly
  Constant1 : Constant  RequirementInfo="{'linktype_rmi_doors' '0000bb43 (/E-STEER Core/SubSystem Specifications/Application Functions/SF99/SF104A Current Regulator Configuration)' '#SF104A_91' 'true' 'REQ:  SF104A_91' '' ; 'linktype_rmi_doors' '0000bb43 (/E-STEER Core/SubSystem Specifications/Application Functions/SF99/SF104A Current Regulator Configuration)' '#SF104A_95' 'true' 'REQ:  SF104A_95' '' } %GIDa_56c3fe74_ffca_4c4a_a539_23b13e41d824"  Value=SysGlbPrmMotPoleCnt
  Constant2 : Constant  RequirementInfo="{'linktype_rmi_doors' '0000bb43 (/E-STEER Core/SubSystem Specifications/Application Functions/SF99/SF104A Current Regulator Configuration)' '#SF104A_95' 'true' 'REQ:  SF104A_95' '' } %GIDa_8a6fb5f9_4b8d_4689_9d54_790a07bee585"  Value=POLETOPHA_ULS_F32  OutDataTypeStr=single
  CopyRight2 : Subsystem  Description=|  mask(Copyright Information){none=on}
      | Copyright info block.                                               
      |                                                                     
      | Place copyright information at the top of every subsystem in design.
      mask prompts: none "No parameters"
      mask help: Place copyright information at the top of every subsystem in design.
      mask Display:
      | NxtrConf = 'Nexteer Confidential';
      | 
      | sys = bdroot; %handle for the current model ("system")
      | first = get_param(sys,'Created');
      | if(isempty(first))
      |     first = datestr(now,'yyyy');
      | else
      |     first = first(end-3:end);  %year is last four digits
      | end
      | 
      | last = get_param(sys,'LastModifiedDate');
      | if isempty(last)
      |     last = datestr(now,'yyyy');
      | else
      |     last = last(end-3:end);
      | end
      | 
      | if strcmp(first,last)
      |     fprintf('%s -- Copyright %s Nexteer',NxtrConf,first)
      | else
      |     fprintf('%s -- %s%s- %s Nexteer',NxtrConf,char(169),first,last)
      | end
  Data Type Conversion : DataTypeConversion  RequirementInfo="{'linktype_rmi_doors' '0000bb43 (/E-STEER Core/SubSystem Specifications/Application Functions/SF99/SF104A Current Regulator Configuration)' '#SF104A_95' 'true' 'REQ:  SF104A_95' '' } %GIDa_842c4066_a436_4475_aeba_ec5c6035272e"  OutDataTypeStr=single
  LimStat_f32 : NxtrLim/LimStat_f32  RequirementInfo="{'linktype_rmi_doors' '0000bb43 (/E-STEER Core/SubSystem Specifications/Application Functions/SF99/SF104A Current Regulator Configuration)' '#SF104A_96' 'true' 'REQ:  SF104A_96' '' } %GIDa_761ed458_7777_41ee_a160_8ceb9a0e1871"  LoLim=MOTAGELECDLYLOLIM_MOTRAD_F32  HiLim=MOTAGELECDLYHILIM_MOTRAD_F32
      settings: AttributesFormatString=|
      | Low Limit: %<LoLim>
      | High Limit:%<HiLim>
  Product : Product  RequirementInfo="{'linktype_rmi_doors' '0000bb43 (/E-STEER Core/SubSystem Specifications/Application Functions/SF99/SF104A Current Regulator Configuration)' '#SF104A_95' 'true' 'REQ:  SF104A_95' '' } %GIDa_5d3b24f5_914b_4689_8f9d_4a5b9b0d275a"  Inputs=3  RndMeth=Zero
  Product1 : Product  RequirementInfo="{'linktype_rmi_doors' '0000bb43 (/E-STEER Core/SubSystem Specifications/Application Functions/SF99/SF104A Current Regulator Configuration)' '#SF104A_95' 'true' 'REQ:  SF104A_95' '' } %GIDa_695e1e92_ecd3_45fd_875b_81368956fd42"
  MotAgElecDly : Outport  RequirementInfo="{'linktype_rmi_doors' '0000bb43 (/E-STEER Core/SubSystem Specifications/Application Functions/SF99/SF104A Current Regulator Configuration)' '#SF104A_95' 'true' 'REQ:  SF104A_95' '' } %GIDa_ff9a667d_1253_49d2_bc27_64b81f3ce83b"
  wires:
  Constant/1 -> Product/2
  Product1/1 -> Product/3
  MotVelMrf/1 -> Product/1
  Product/1 -> LimStat_f32/1
  Constant1/1 -> Data Type Conversion/1
  Constant2/1 -> Product1/2
  Data Type Conversion/1 -> Product1/1
  LimStat_f32/1 -> MotAgElecDly/1

== system SF104A_MotCurrRegCfg/MotCurrRegCfg/MotCurrRegCfgPer1/CopyRight2 ==

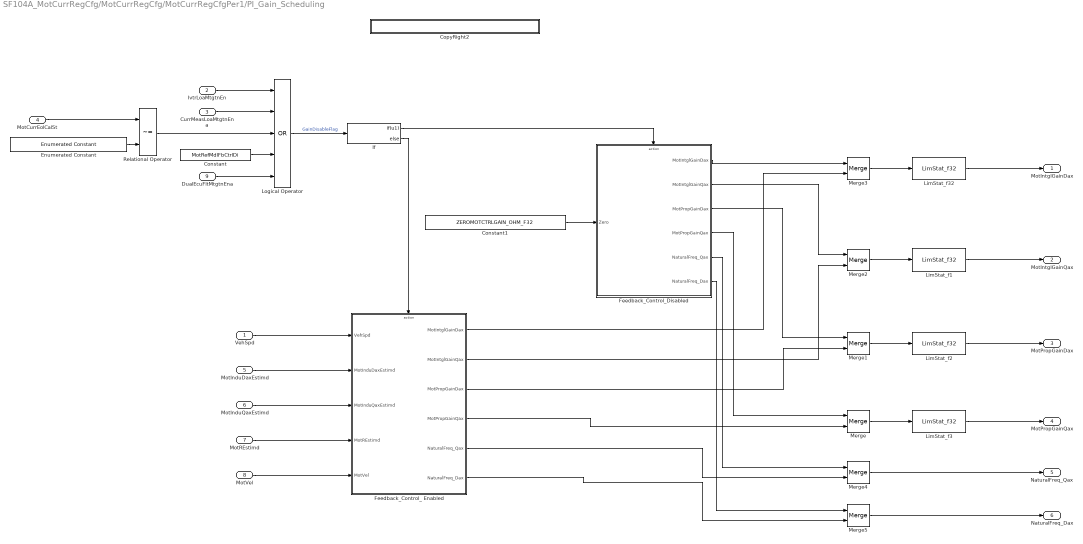
== system SF104A_MotCurrRegCfg/MotCurrRegCfg/MotCurrRegCfgPer1/PI_Gain_Scheduling ==
  VehSpd : Inport
  IvtrLoaMtgtnEn : Inport  RequirementInfo="{'linktype_rmi_doors' '0000bb43 (/E-STEER Core/SubSystem Specifications/Application Functions/SF99/SF104A Current Regulator Configuration)' '#SF104A_84' 'true' 'REQ:  SF104A_84' '' } %GIDa_bffe6544_874e_4981_88f5_1a4fe8d4cae5"  Port=2
  CurrMeasLoaMtgtnEna : Inport  RequirementInfo="{'linktype_rmi_doors' '0000bb43 (/E-STEER Core/SubSystem Specifications/Application Functions/SF99/SF104A Current Regulator Configuration)' '#SF104A_84' 'true' 'REQ:  SF104A_84' '' } %GIDa_d871df1c_d382_4087_b45a_c19450a0507f"  Port=3
  MotCurrEolCalSt : Inport  RequirementInfo="{'linktype_rmi_doors' '0000bb43 (/E-STEER Core/SubSystem Specifications/Application Functions/SF99/SF104A Current Regulator Configuration)' '#SF104A_84' 'true' 'REQ:  SF104A_84' '' } %GIDa_7ae90866_0438_4d9f_abcf_c257559127dd"  Port=4
  MotInduDaxEstimd : Inport  Port=5
  MotInduQaxEstimd : Inport  Port=6
  MotREstimd : Inport  Port=7
  MotVel : Inport  Port=8
  DualEcuFltMtgtnEna : Inport  RequirementInfo="{'linktype_rmi_doors' '0000bb43 (/E-STEER Core/SubSystem Specifications/Application Functions/SF99/SF104A Current Regulator Configuration)' '#SF104A_44' 'true' 'REQ:  SF104A_44' '' } %GIDa_f5a72bff_4bed_4314_976e_7581af6ad4fe"  Port=9
  Constant : Constant  RequirementInfo="{'linktype_rmi_doors' '0000bb43 (/E-STEER Core/SubSystem Specifications/Application Functions/SF99/SF104A Current Regulator Configuration)' '#SF104A_84' 'true' 'REQ:  SF104A_84' '' } %GIDa_d491614a_9929_44f6_aa9e_e33a954a26bd"  Value=MotRefMdlFbCtrlDi
  Constant1 : Constant  RequirementInfo="{'linktype_rmi_doors' '0000bb43 (/E-STEER Core/SubSystem Specifications/Application Functions/SF99/SF104A Current Regulator Configuration)' '#SF104A_85' 'true' 'REQ:  SF104A_85' '' } %GIDa_656dea14_7db3_4d24_9d38_794349feffd4"  Value=ZEROMOTCTRLGAIN_OHM_F32  OutDataTypeStr=single
  CopyRight2 : Subsystem  Description=|  mask(Copyright Information){none=on}
      | Copyright info block.                                               
      |                                                                     
      | Place copyright information at the top of every subsystem in design.
      mask prompts: none "No parameters"
      mask help: Place copyright information at the top of every subsystem in design.
      mask Display:
      | NxtrConf = 'Nexteer Confidential';
      | 
      | sys = bdroot; %handle for the current model ("system")
      | first = get_param(sys,'Created');
      | if(isempty(first))
      |     first = datestr(now,'yyyy');
      | else
      |     first = first(end-3:end);  %year is last four digits
      | end
      | 
      | last = get_param(sys,'LastModifiedDate');
      | if isempty(last)
      |     last = datestr(now,'yyyy');
      | else
      |     last = last(end-3:end);
      | end
      | 
      | if strcmp(first,last)
      |     fprintf('%s -- Copyright %s Nexteer',NxtrConf,first)
      | else
      |     fprintf('%s -- %s%s- %s Nexteer',NxtrConf,char(169),first,last)
      | end
  Enumerated Constant : simulink/Sources/Enumerated Constant  RequirementInfo="{'linktype_rmi_doors' '0000bb43 (/E-STEER Core/SubSystem Specifications/Application Functions/SF99/SF104A Current Regulator Configuration)' '#SF104A_84' 'true' 'REQ:  SF104A_84' '' } %GIDa_e7125504_1e4e_4a29_9eda_664ececb0e0e"  OutDataTypeStr=Enum: MotCurrEolCalSt2  Value=MotCurrEolCalSt2.MCECS_OFFSCMDSTRT  SampleTime=inf
  Feedback_Control_ Enabled : Subsystem  TreatAsAtomicUnit=on
  Feedback_Control_Disabled : Subsystem  RequirementInfo="{'linktype_rmi_doors' '0000bb43 (/E-STEER Core/SubSystem Specifications/Application Functions/SF99/SF104A Current Regulator Configuration)' '#SF104A_85' 'true' 'REQ:  SF104A_85' '' } %GIDa_a9ff782d_19a4_4b75_a613_5de15ede7554"  TreatAsAtomicUnit=on
      settings: AttributesFormatString=pass_thru only
  If : If  RequirementInfo="{'linktype_rmi_doors' '0000bb43 (/E-STEER Core/SubSystem Specifications/Application Functions/SF99/SF104A Current Regulator Configuration)' '#SF104A_85' 'true' 'REQ:  SF104A_85' '' } %GIDa_abc8314a_4171_41fa_8bec_9fbb25de47f4"  IfExpression=u1
  LimStat_f1 : NxtrLim/LimStat_f32  RequirementInfo="{'linktype_rmi_doors' '0000bb43 (/E-STEER Core/SubSystem Specifications/Application Functions/SF99/SF104A Current Regulator Configuration)' '#SF104A_96' 'true' 'REQ:  SF104A_96' '' } %GIDa_b3887a97_c2c9_41d6_b6c6_33417ab411f9"  LoLim=MOTINTGLGAINLOLIM_OHM_F32  HiLim=MOTINTGLGAINHILIM_OHM_F32
      settings: AttributesFormatString=|
      | Low Limit: %<LoLim>
      | High Limit:%<HiLim>
  LimStat_f2 : NxtrLim/LimStat_f32  RequirementInfo="{'linktype_rmi_doors' '0000bb43 (/E-STEER Core/SubSystem Specifications/Application Functions/SF99/SF104A Current Regulator Configuration)' '#SF104A_96' 'true' 'REQ:  SF104A_96' '' } %GIDa_7b3aa5d0_fee3_47c1_ba90_de323ff22edb"  LoLim=MOTPROPGAINLOLIM_OHM_F32  HiLim=MOTPROPGAINHILIM_OHM_F32
      settings: AttributesFormatString=|
      | Low Limit: %<LoLim>
      | High Limit:%<HiLim>
  LimStat_f3 : NxtrLim/LimStat_f32  RequirementInfo="{'linktype_rmi_doors' '0000bb43 (/E-STEER Core/SubSystem Specifications/Application Functions/SF99/SF104A Current Regulator Configuration)' '#SF104A_96' 'true' 'REQ:  SF104A_96' '' } %GIDa_41f66751_a2fa_46ce_8361_435cfda7cbfd"  LoLim=MOTPROPGAINLOLIM_OHM_F32  HiLim=MOTPROPGAINHILIM_OHM_F32
      settings: AttributesFormatString=|
      | Low Limit: %<LoLim>
      | High Limit:%<HiLim>
  LimStat_f32 : NxtrLim/LimStat_f32  RequirementInfo="{'linktype_rmi_doors' '0000bb43 (/E-STEER Core/SubSystem Specifications/Application Functions/SF99/SF104A Current Regulator Configuration)' '#SF104A_96' 'true' 'REQ:  SF104A_96' '' } %GIDa_a7ad6de3_dada_42e2_9534_937e985b6a5b"  LoLim=MOTINTGLGAINLOLIM_OHM_F32  HiLim=MOTINTGLGAINHILIM_OHM_F32
      settings: AttributesFormatString=|
      | Low Limit: %<LoLim>
      | High Limit:%<HiLim>
  Logical Operator : Logic  RequirementInfo="{'linktype_rmi_doors' '0000bb43 (/E-STEER Core/SubSystem Specifications/Application Functions/SF99/SF104A Current Regulator Configuration)' '#SF104A_84' 'true' 'REQ:  SF104A_84' '' } %GIDa_89f7dedb_df01_4607_95b8_da4cee3a47fb"  Operator=OR  Inputs=5  AllPortsSameDT=off  OutDataTypeStr=boolean
  Merge{,1..5} (6 alike) : Merge
  Relational Operator : RelationalOperator  RequirementInfo="{'linktype_rmi_doors' '0000bb43 (/E-STEER Core/SubSystem Specifications/Application Functions/SF99/SF104A Current Regulator Configuration)' '#SF104A_84' 'true' 'REQ:  SF104A_84' '' } %GIDa_ab6b1f6c_1568_4502_91c9_85719c8a373f"  Operator=~=  OutDataTypeStr=boolean
  MotIntglGainDax : Outport
  MotIntglGainQax : Outport  Port=2
  MotPropGainDax : Outport  Port=3
  MotPropGainQax : Outport  Port=4
  NaturalFreq_Qax : Outport  Port=5
  NaturalFreq_Dax : Outport  Port=6
  wires:
  IvtrLoaMtgtnEn/1 -> Logical Operator/1
  CurrMeasLoaMtgtnEna/1 -> Logical Operator/2
  Constant/1 -> Logical Operator/4
  MotCurrEolCalSt/1 -> Relational Operator/1
  Enumerated Constant/1 -> Relational Operator/2
  Relational Operator/1 -> Logical Operator/3
  Logical Operator/1 -> If/1  "GainDisableFlag"
  If/1 -> Feedback_Control_Disabled/Action
  Constant1/1 -> Feedback_Control_Disabled/1(Zero)
  If/2 -> Feedback_Control_ Enabled/Action
  VehSpd/1 -> Feedback_Control_ Enabled/1(VehSpd)
  MotInduQaxEstimd/1 -> Feedback_Control_ Enabled/3(MotInduQaxEstimd)
  MotVel/1 -> Feedback_Control_ Enabled/5(MotVel)
  MotInduDaxEstimd/1 -> Feedback_Control_ Enabled/2(MotInduDaxEstimd)
  MotREstimd/1 -> Feedback_Control_ Enabled/4(MotREstimd)
  Feedback_Control_ Enabled/5(NaturalFreq_Qax) -> Merge4/2
  Feedback_Control_ Enabled/6(NaturalFreq_Dax) -> Merge5/2
  Feedback_Control_ Enabled/4(MotPropGainQax) -> Merge/2
  Feedback_Control_ Enabled/3(MotPropGainDax) -> Merge1/2
  Feedback_Control_ Enabled/2(MotIntglGainQax) -> Merge2/2
  Feedback_Control_ Enabled/1(MotIntglGainDax) -> Merge3/2
  Feedback_Control_Disabled/4(MotPropGainQax) -> Merge/1
  Feedback_Control_Disabled/3(MotPropGainDax) -> Merge1/1
  Feedback_Control_Disabled/2(MotIntglGainQax) -> Merge2/1
  Feedback_Control_Disabled/1(MotIntglGainDax) -> Merge3/1
  Merge3/1 -> LimStat_f32/1
  Merge2/1 -> LimStat_f1/1
  Merge1/1 -> LimStat_f2/1
  Merge/1 -> LimStat_f3/1
  LimStat_f32/1 -> MotIntglGainDax/1
  LimStat_f1/1 -> MotIntglGainQax/1
  LimStat_f2/1 -> MotPropGainDax/1
  LimStat_f3/1 -> MotPropGainQax/1
  Feedback_Control_Disabled/5(NaturalFreq_Qax) -> Merge4/1
  Feedback_Control_Disabled/6(NaturalFreq_Dax) -> Merge5/1
  Merge4/1 -> NaturalFreq_Qax/1
  Merge5/1 -> NaturalFreq_Dax/1
  DualEcuFltMtgtnEna/1 -> Logical Operator/5

== system SF104A_MotCurrRegCfg/MotCurrRegCfg/MotCurrRegCfgPer1/2nd_Order_Damping_Terms/CopyRight2 ==

== system SF104A_MotCurrRegCfg/MotCurrRegCfg/MotCurrRegCfgPer1/Calc MotAgElecDly/CopyRight2 ==

== system SF104A_MotCurrRegCfg/MotCurrRegCfg/MotCurrRegCfgPer1/PI_Gain_Scheduling/CopyRight2 ==
